simulink model "invpend"  (R2024b)
settings: Solver=VariableStepAuto  StartTime=0.0  StopTime=20  RelTol=1e-3
values from neighbouring files (symbols this model uses):
  b = []    [autoQR.m]
  g = 9.81    [robot.m]    (also in robot_cascade.m; robot_linear.m; robot_lqr.m)
  l = 0.08    [robot.m]    (also in robot_cascade.m; robot_linear.m)
  m = 0.33    [robot.m]    (also in robot_cascade.m; robot_linear.m; robot_lqr.m)
  M = 1.180    (= 1.18)    [robot.m]    (also in robot_cascade.m; robot_linear.m; robot_lqr.m)
undefined symbols (not defined in the file or in its folder): I
settings Model: Creator=cosr3  LastModifiedBy=cosr3

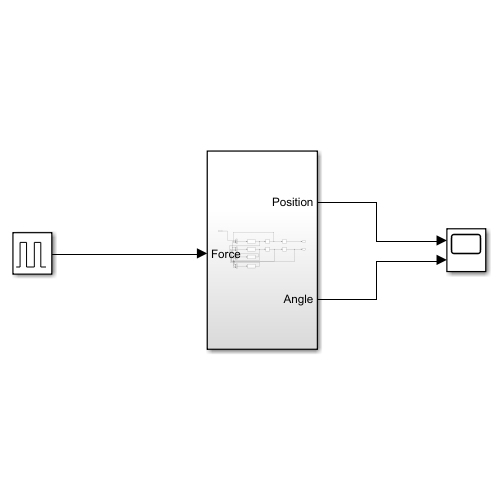
[thumbnail: Simulink's stored preview of the top-level diagram]
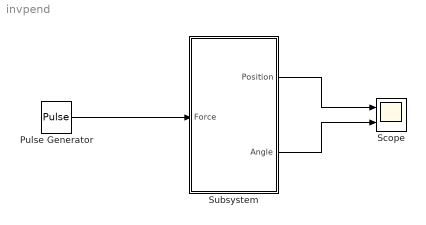
== system invpend ==
  Pulse Generator : DiscretePulseGenerator  PulseType=Time based  Period=10  PulseWidth=5
  Scope : Scope  NumInputPorts=2
  Subsystem : Subsystem
  wires:
  Pulse Generator/1 -> Subsystem/1(Force)
  Subsystem/1(Position) -> Scope/1
  Subsystem/2(Angle) -> Scope/2

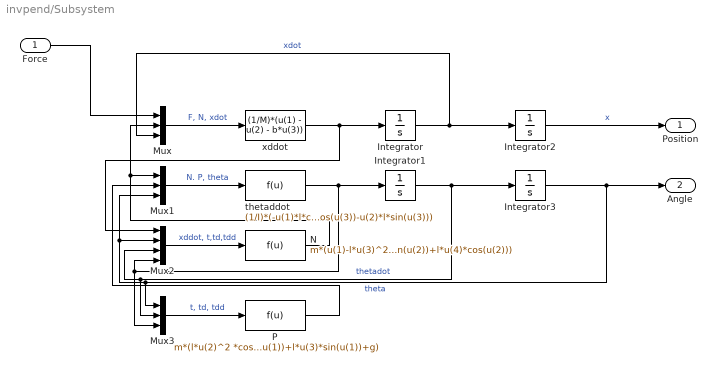
== system invpend/Subsystem ==
  Force : Inport
  Integrator : Integrator  ContinuousStateAttributes='xdot'
  Integrator1 : Integrator  InitialCondition=pi  ContinuousStateAttributes='thetadot'
  Integrator2 : Integrator  ContinuousStateAttributes='x'
  Integrator3 : Integrator  ContinuousStateAttributes='theta'
  Mux : Mux  Inputs=3
  Mux1 : Mux  Inputs=3
  Mux2 : Mux
  Mux3 : Mux  Inputs=3
  N : Fcn  Expr=m*(u(1)-l*u(3)^2*sin(u(2))+l*u(4)*cos(u(2)))
  P : Fcn  Expr=m*(l*u(2)^2 *cos(u(1))+l*u(3)*sin(u(1))+g)
  thetaddot : Fcn  Expr=(1/I)*(-u(1)*l*cos(u(3))-u(2)*l*sin(u(3)))
  xddot : Fcn  Expr=(1/M)*(u(1) - u(2) - b*u(3))
  Position : Outport
  Angle : Outport  Port=2
  wires:
  xddot/1 -> Mux2/1, Integrator/1
  thetaddot/1 -> Mux3/3, Mux2/4, Integrator1/1
  Mux2/1 -> N/1  "xddot, t,td,tdd"
  Integrator2/1 -> Position/1  "x"
  Force/1 -> Mux/1
  Integrator/1 -> Mux/3, Integrator2/1  "xdot"
  Mux1/1 -> thetaddot/1  "N. P, theta"
  Integrator3/1 -> Angle/1, Mux3/1, Mux2/2, Mux1/3  "theta"
  Mux3/1 -> P/1  "t, td, tdd"
  Integrator1/1 -> Mux3/2, Mux2/3, Integrator3/1  "thetadot"
  Mux/1 -> xddot/1  "F, N, xdot"
  N/1 -> Mux/2, Mux1/1
  P/1 -> Mux1/2
